simulink model "Chiari"  (R2024b)
settings: Solver=FixedStepAuto  StartTime=0.0  StopTime=60  FixedStep=0.05  RelTol=1e-3
settings Model: Creator=dossantos  LastModifiedBy=dossantos

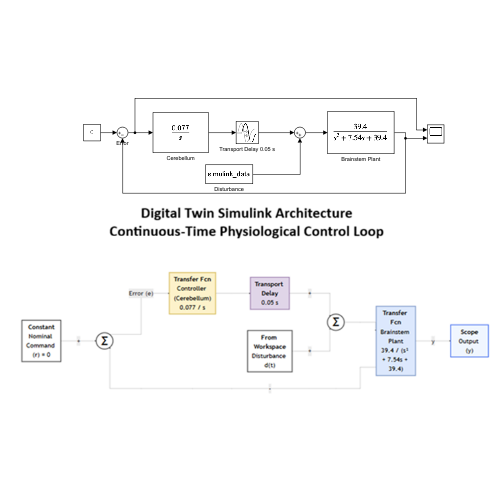
[thumbnail: Simulink's stored preview of the top-level diagram]
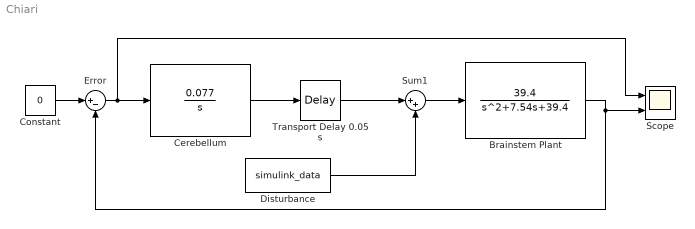
== system Chiari ==
  Brainstem Plant : TransferFcn  Numerator=[39.4]  Denominator=[1 7.54 39.4]
  Cerebellum : TransferFcn  Numerator=[0.077]  Denominator=[1 0]
  Constant : Constant  Value=0
  Disturbance : FromWorkspace  VariableName=simulink_data  SampleTime=0.05  Interpolate=off  OutputAfterFinalValue=Cyclic repetition
  Error : Sum  Inputs=|+-
  Scope : Scope  NumInputPorts=2
  Sum1 : Sum  Inputs=|++
  Transport Delay 0.05 s : TransportDelay  DelayTime=0.05
  wires:
  Constant/1 -> Error/1
  Brainstem Plant/1 -> Error/2, Scope/2
  Cerebellum/1 -> Transport Delay 0.05 s/1
  Transport Delay 0.05 s/1 -> Sum1/1
  Sum1/1 -> Brainstem Plant/1
  Disturbance/1 -> Sum1/2
  Error/1 -> Scope/1, Cerebellum/1
